simulink model "gm_fourxfour_designfxdpt_givens"  (R2018b)
settings: Solver=FixedStepDiscrete  StartTime=0.0  StopTime=0.18e-6  RelTol=1e-3
InitFcn:
  | if isempty(which('mylib'))
  |      tmp = fileparts(which(bdroot));
  |      run(fullfile(fileparts(tmp), '5-Utilities', 'addPathsPfcHw.m'));
  | end
  | 
  | data_types_givens
StopFcn:
  | GivensSim_Stop
undefined symbols (not defined in the file or in its folder): f
(part 1 of 3)
settings Model: Creator=skanaga4  LastModifiedBy=yangli18
settings OptimizationCC: BlockReduction=off  ConditionallyExecuteInputs=off  DefaultParameterBehavior=Inlined
settings DebuggingCC: AlgebraicLoopMsg=error  ArtificialAlgebraicLoopMsg=none  InheritedTsInSrcMsg=none  SingleTaskRateTransMsg=error
settings HardwareCC: ProdBitPerPointer=32  ProdBitPerSizeT=32  ProdBitPerPtrDiffT=32  ProdLargestAtomicFloat=None  ProdIntDivRoundTo=Undefined  ProdEndianess=Unspecified  ProdWordSize=32  ProdHWDeviceType=ASIC/FPGA->ASIC/FPGA  TargetBitPerLong=64  TargetBitPerPointer=64  TargetBitPerSizeT=64  TargetBitPerPtrDiffT=64  TargetLongLongMode=on  TargetIntDivRoundTo=Zero  TargetEndianess=LittleEndian  TargetWordSize=64  TargetHWDeviceType=Custom Processor->MATLAB Host Computer  ProdEqTarget=off

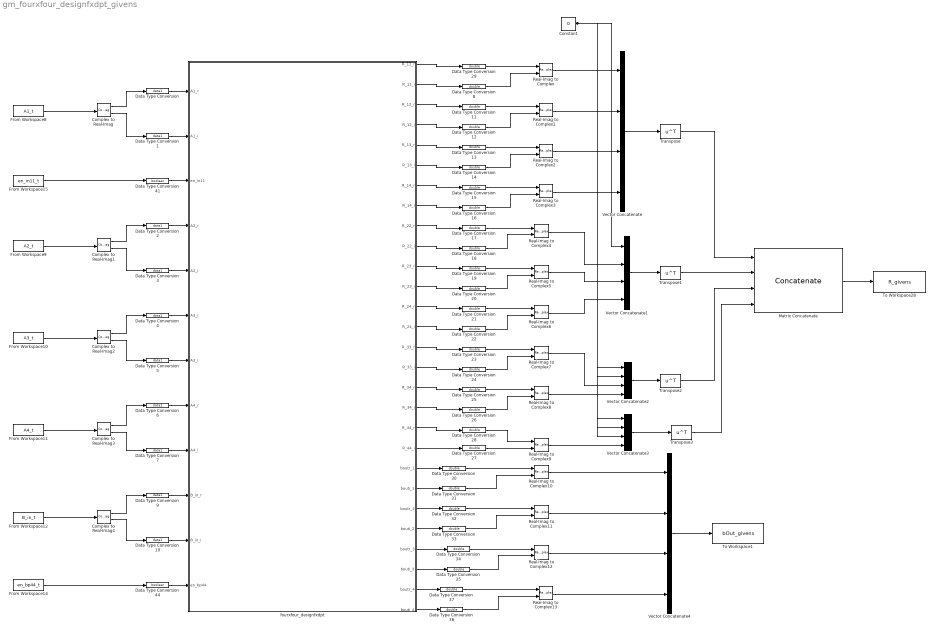
== system gm_fourxfour_designfxdpt_givens ==
  Complex to Real-Imag{,1..4} (5 alike) : ComplexToRealImag
  Constant : Constant  Value=0  SampleTime=-1
  Data Type Conversion{,1..7,9..10} (10 alike) : DataTypeConversion  OutDataTypeStr=data1
  Data Type Conversion{8,11..37} (28 alike) : DataTypeConversion  OutDataTypeStr=double
  Data Type Conversion41 : DataTypeConversion  OutDataTypeStr=boolean
  Data Type Conversion44 : DataTypeConversion  OutDataTypeStr=boolean
  From Workspace10 : FromWorkspace  VariableName=A3_t  SampleTime=1/f  Interpolate=off  OutputAfterFinalValue=Holding final value
  From Workspace11 : FromWorkspace  VariableName=A4_t  SampleTime=1/f  Interpolate=off  OutputAfterFinalValue=Holding final value
  From Workspace12 : FromWorkspace  VariableName=B_in_t  SampleTime=1/f  Interpolate=off  OutputAfterFinalValue=Holding final value
  From Workspace14 : FromWorkspace  VariableName=en_bp44_t  SampleTime=1/f  Interpolate=off  OutputAfterFinalValue=Holding final value
  From Workspace15 : FromWorkspace  VariableName=en_in11_t  SampleTime=1/f  Interpolate=off  OutputAfterFinalValue=Holding final value
  From Workspace8 : FromWorkspace  VariableName=A1_t  SampleTime=1/f  Interpolate=off  OutputAfterFinalValue=Holding final value
  From Workspace9 : FromWorkspace  VariableName=A2_t  SampleTime=1/f  Interpolate=off  OutputAfterFinalValue=Holding final value
  Matrix Concatenate : Concatenate  NumInputs=4  Mode=Multidimensional array
  Real-Imag to Complex{,1..13} (14 alike) : RealImagToComplex
  To Workspace1 : ToWorkspace  VariableName=bOut_givens  SaveFormat=Timeseries  SampleTime=-1
  To Workspace28 : ToWorkspace  VariableName=R_givens  SaveFormat=Timeseries  SampleTime=-1
  Transpose{,1..3} (4 alike) : Math  Operator=transpose  RndMeth=Zero  SaturateOnIntegerOverflow=on
  Vector Concatenate{,1..4} (5 alike) : Concatenate  NumInputs=4
  fourxfour_designfxdpt : Subsystem
  wires:
  Vector Concatenate4/1 -> To Workspace1/1
  Real-Imag to Complex13/1 -> Vector Concatenate4/4
  Real-Imag to Complex12/1 -> Vector Concatenate4/3
  Data Type Conversion30/1 -> Real-Imag to Complex10/1
  Data Type Conversion37/1 -> Real-Imag to Complex13/1
  Data Type Conversion32/1 -> Real-Imag to Complex11/1
  Data Type Conversion33/1 -> Real-Imag to Complex11/2
  Data Type Conversion34/1 -> Real-Imag to Complex12/1
  Real-Imag to Complex11/1 -> Vector Concatenate4/2
  Real-Imag to Complex10/1 -> Vector Concatenate4/1
  Data Type Conversion31/1 -> Real-Imag to Complex10/2
  Data Type Conversion35/1 -> Real-Imag to Complex12/2
  Data Type Conversion36/1 -> Real-Imag to Complex13/2
  fourxfour_designfxdpt/14(R_24_i) -> Data Type Conversion22/1
  fourxfour_designfxdpt/15(R_33_r) -> Data Type Conversion23/1
  fourxfour_designfxdpt/16(R_33_i) -> Data Type Conversion24/1
  fourxfour_designfxdpt/17(R_34_r) -> Data Type Conversion25/1
  fourxfour_designfxdpt/18(R_34_i) -> Data Type Conversion26/1
  Data Type Conversion27/1 -> Real-Imag to Complex9/2
  fourxfour_designfxdpt/19(R_44_r) -> Data Type Conversion28/1
  Real-Imag to Complex3/1 -> Vector Concatenate/4
  Data Type Conversion14/1 -> Real-Imag to Complex2/2
  Real-Imag to Complex1/1 -> Vector Concatenate/2
  Data Type Conversion11/1 -> Real-Imag to Complex1/1
  Data Type Conversion26/1 -> Real-Imag to Complex8/2
  Vector Concatenate2/1 -> Transpose2/1
  Data Type Conversion22/1 -> Real-Imag to Complex6/2
  fourxfour_designfxdpt/10(R_22_i) -> Data Type Conversion18/1
  fourxfour_designfxdpt/1(R_11_r) -> Data Type Conversion29/1
  Transpose1/1 -> Matrix Concatenate/2
  fourxfour_designfxdpt/11(R_23_r) -> Data Type Conversion19/1
  Real-Imag to Complex6/1 -> Vector Concatenate1/4
  Vector Concatenate1/1 -> Transpose1/1
  fourxfour_designfxdpt/20(R_44_i) -> Data Type Conversion27/1
  Data Type Conversion20/1 -> Real-Imag to Complex5/2
  Transpose2/1 -> Matrix Concatenate/3
  Data Type Conversion19/1 -> Real-Imag to Complex5/1
  fourxfour_designfxdpt/8(R_14_i) -> Data Type Conversion16/1
  fourxfour_designfxdpt/13(R_24_r) -> Data Type Conversion21/1
  Transpose3/1 -> Matrix Concatenate/4
  fourxfour_designfxdpt/9(R_22_r) -> Data Type Conversion17/1
  Real-Imag to Complex7/1 -> Vector Concatenate2/3
  fourxfour_designfxdpt/2(R_11_i) -> Data Type Conversion8/1
  Transpose/1 -> Matrix Concatenate/1
  fourxfour_designfxdpt/12(R_23_i) -> Data Type Conversion20/1
  Data Type Conversion25/1 -> Real-Imag to Complex8/1
  Data Type Conversion24/1 -> Real-Imag to Complex7/2
  Data Type Conversion8/1 -> Real-Imag to Complex/2
  Data Type Conversion23/1 -> Real-Imag to Complex7/1
  fourxfour_designfxdpt/7(R_14_r) -> Data Type Conversion15/1
  Vector Concatenate3/1 -> Transpose3/1
  fourxfour_designfxdpt/5(R_13_r) -> Data Type Conversion13/1
  fourxfour_designfxdpt/4(R_12_i) -> Data Type Conversion12/1
  fourxfour_designfxdpt/3(R_12_r) -> Data Type Conversion11/1
  fourxfour_designfxdpt/6(R_13_i) -> Data Type Conversion14/1
  Matrix Concatenate/1 -> To Workspace28/1
  Data Type Conversion29/1 -> Real-Imag to Complex/1
  Data Type Conversion28/1 -> Real-Imag to Complex9/1
  Data Type Conversion15/1 -> Real-Imag to Complex3/1
  Data Type Conversion18/1 -> Real-Imag to Complex4/2
  Data Type Conversion17/1 -> Real-Imag to Complex4/1
  Data Type Conversion16/1 -> Real-Imag to Complex3/2
  Data Type Conversion12/1 -> Real-Imag to Complex1/2
  Data Type Conversion13/1 -> Real-Imag to Complex2/1
  Data Type Conversion21/1 -> Real-Imag to Complex6/1
  Real-Imag to Complex5/1 -> Vector Concatenate1/3
  Vector Concatenate/1 -> Transpose/1
  Real-Imag to Complex2/1 -> Vector Concatenate/3
  Real-Imag to Complex8/1 -> Vector Concatenate2/4
  Real-Imag to Complex9/1 -> Vector Concatenate3/4
  Real-Imag to Complex4/1 -> Vector Concatenate1/2
  Constant/1 -> Vector Concatenate1/1, Vector Concatenate2/1, Vector Concatenate2/2, Vector Concatenate3/1, Vector Concatenate3/2, Vector Concatenate3/3
  Real-Imag to Complex/1 -> Vector Concatenate/1
  From Workspace15/1 -> Data Type Conversion41/1
  From Workspace14/1 -> Data Type Conversion44/1
  Complex to Real-Imag4/2 -> Data Type Conversion10/1
  Complex to Real-Imag4/1 -> Data Type Conversion9/1
  From Workspace12/1 -> Complex to Real-Imag4/1
  Complex to Real-Imag3/2 -> Data Type Conversion7/1
  Complex to Real-Imag3/1 -> Data Type Conversion6/1
  Complex to Real-Imag2/2 -> Data Type Conversion5/1
  Complex to Real-Imag2/1 -> Data Type Conversion4/1
  Complex to Real-Imag1/2 -> Data Type Conversion3/1
  Complex to Real-Imag1/1 -> Data Type Conversion2/1
  From Workspace10/1 -> Complex to Real-Imag2/1
  From Workspace11/1 -> Complex to Real-Imag3/1
  From Workspace9/1 -> Complex to Real-Imag1/1
  Complex to Real-Imag/2 -> Data Type Conversion1/1
  Complex to Real-Imag/1 -> Data Type Conversion/1
  From Workspace8/1 -> Complex to Real-Imag/1
  Data Type Conversion10/1 -> fourxfour_designfxdpt/11(B_in_i)
  Data Type Conversion9/1 -> fourxfour_designfxdpt/10(B_in_r)
  fourxfour_designfxdpt/26(bouti_3) -> Data Type Conversion35/1
  fourxfour_designfxdpt/25(boutr_3) -> Data Type Conversion34/1
  fourxfour_designfxdpt/27(boutr_4) -> Data Type Conversion37/1
  fourxfour_designfxdpt/28(bouti_4) -> Data Type Conversion36/1
  fourxfour_designfxdpt/23(boutr_2) -> Data Type Conversion32/1
  fourxfour_designfxdpt/24(bouti_2) -> Data Type Conversion33/1
  fourxfour_designfxdpt/22(bouti_1) -> Data Type Conversion31/1
  fourxfour_designfxdpt/21(boutr_1) -> Data Type Conversion30/1
  Data Type Conversion44/1 -> fourxfour_designfxdpt/12(en_bp44)
  Data Type Conversion41/1 -> fourxfour_designfxdpt/3("en_in11 ")
  Data Type Conversion7/1 -> fourxfour_designfxdpt/9(A4_i)
  Data Type Conversion6/1 -> fourxfour_designfxdpt/8(A4_r)
  Data Type Conversion5/1 -> fourxfour_designfxdpt/7(A3_i)
  Data Type Conversion4/1 -> fourxfour_designfxdpt/6(A3_r)
  Data Type Conversion3/1 -> fourxfour_designfxdpt/5(A2_i)
  Data Type Conversion2/1 -> fourxfour_designfxdpt/4(A2_r)
  Data Type Conversion1/1 -> fourxfour_designfxdpt/2(A1_i)
  Data Type Conversion/1 -> fourxfour_designfxdpt/1("A1_r ")

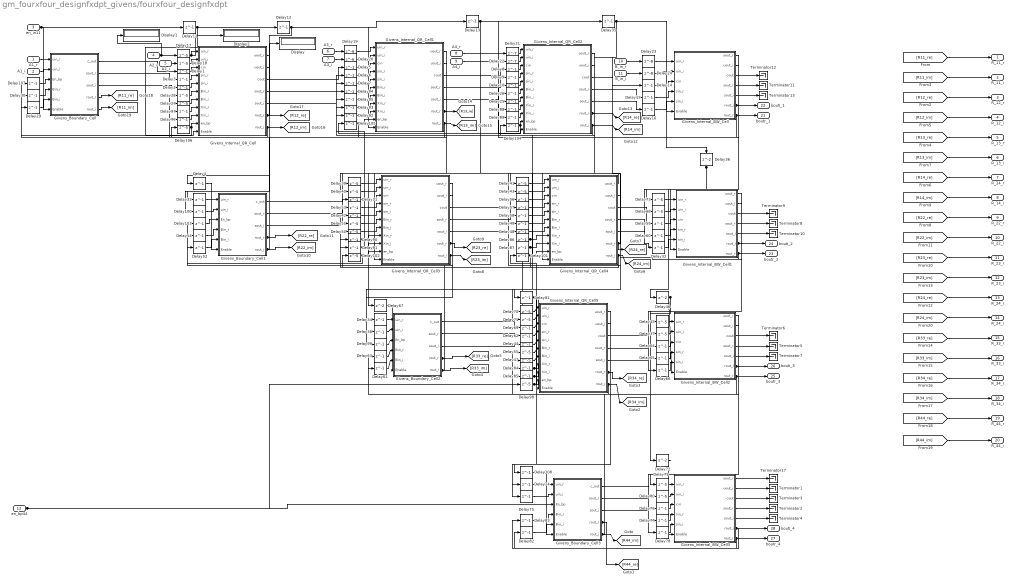
== system gm_fourxfour_designfxdpt_givens/fourxfour_designfxdpt ==
  "A1_r " : Inport  OutDataTypeStr=fixdt(1, 24, 14)  PortDimensions=1  SampleTime=1e-08
  A1_i : Inport  Port=2  OutDataTypeStr=fixdt(1, 24, 14)  PortDimensions=1  SampleTime=1e-08
  "en_in11 " : Inport  Port=3  OutDataTypeStr=boolean  PortDimensions=1  SampleTime=1e-08
  A2_r : Inport  Port=4  OutDataTypeStr=fixdt(1, 24, 14)  PortDimensions=1  SampleTime=1e-08
  A2_i : Inport  Port=5  OutDataTypeStr=fixdt(1, 24, 14)  PortDimensions=1  SampleTime=1e-08
  A3_r : Inport  Port=6  OutDataTypeStr=fixdt(1, 24, 14)  PortDimensions=1  SampleTime=1e-08
  A3_i : Inport  Port=7  OutDataTypeStr=fixdt(1, 24, 14)  PortDimensions=1  SampleTime=1e-08
  A4_r : Inport  Port=8  OutDataTypeStr=fixdt(1, 24, 14)  PortDimensions=1  SampleTime=1e-08
  A4_i : Inport  Port=9  OutDataTypeStr=fixdt(1, 24, 14)  PortDimensions=1  SampleTime=1e-08
  B_in_r : Inport  Port=10  OutDataTypeStr=fixdt(1, 24, 14)  PortDimensions=1  SampleTime=1e-08
  B_in_i : Inport  Port=11  OutDataTypeStr=fixdt(1, 24, 14)  PortDimensions=1  SampleTime=1e-08
  en_bp44 : Inport  Port=12  OutDataTypeStr=boolean  PortDimensions=1  SampleTime=1e-08
  Delay{1..16,25..26,29..35,38,42,44,48..49,52..54,56..66,69,74..78,81..97,99..101,103..105,107..108} (75 alike) : Delay  DelayLength=1  InitialCondition=0
  Delay{17..18,27..28,37,39..41,43,45,47,50..51,55,68,70..71,73,79..80,98,102,106} (23 alike) : Delay  DelayLength=5  InitialCondition=0
  Delay19 : Delay  DelayLength=6  InitialCondition=0
  Delay20 : Delay  DelayLength=6  InitialCondition=0
  Delay21 : Delay  DelayLength=7  InitialCondition=0
  Delay22 : Delay  DelayLength=7  InitialCondition=0
  Delay23 : Delay  DelayLength=8  InitialCondition=0
  Delay24 : Delay  DelayLength=8  InitialCondition=0
  Delay{36,46,67,72} (4 alike) : Delay  InitialCondition=0
  Display : Display
  Display1 : Display
  Display2 : Display
  Givens_Boundary_Cell : Subsystem
  Givens_Boundary_Cell1 : Subsystem
  Givens_Boundary_Cell2 : Subsystem
  Givens_Boundary_Cell3 : Subsystem
  Givens_Internal_BW_Cell : Subsystem
  Givens_Internal_BW_Cell1 : Subsystem
  Givens_Internal_BW_Cell2 : Subsystem
  Givens_Internal_BW_Cell3 : Subsystem
  Givens_Internal_QR_Cell : Subsystem
  Givens_Internal_QR_Cell1 : Subsystem
  Givens_Internal_QR_Cell2 : Subsystem
  Givens_Internal_QR_Cell3 : Subsystem
  Givens_Internal_QR_Cell4 : Subsystem
  Givens_Internal_QR_Cell5 : Subsystem
  Terminator{1..13,17} (14 alike) : Terminator
  R_11_r : Outport
  R_11_i : Outport  Port=2
  R_12_r : Outport  Port=3
  R_12_i : Outport  Port=4
  R_13_r : Outport  Port=5
  R_13_i : Outport  Port=6
  R_14_r : Outport  Port=7
  R_14_i : Outport  Port=8
  R_22_r : Outport  Port=9
  R_22_i : Outport  Port=10
  R_23_r : Outport  Port=11
  R_23_i : Outport  Port=12
  R_24_r : Outport  Port=13
  R_24_i : Outport  Port=14
  R_33_r : Outport  Port=15
  R_33_i : Outport  Port=16
  R_34_r : Outport  Port=17
  R_34_i : Outport  Port=18
  R_44_r : Outport  Port=19
  R_44_i : Outport  Port=20
  boutr_1 : Outport  Port=21
  bouti_1 : Outport  Port=22
  boutr_2 : Outport  Port=23
  bouti_2 : Outport  Port=24
  boutr_3 : Outport  Port=25
  bouti_3 : Outport  Port=26
  boutr_4 : Outport  Port=27
  bouti_4 : Outport  Port=28
  wires:
  "A1_r "/1 -> Givens_Boundary_Cell/1(uin_r)
  A1_i/1 -> Givens_Boundary_Cell/2(uin_i)
  "en_in11 "/1 -> Delay11/1, Givens_Boundary_Cell/6(Enable)
  A2_r/1 -> Display1/1, Delay17/1
  A2_i/1 -> Delay18/1
  A3_r/1 -> Delay19/1
  A3_i/1 -> Delay20/1
  A4_r/1 -> Delay21/1
  A4_i/1 -> Delay22/1
  B_in_r/1 -> Delay23/1
  B_in_i/1 -> Delay24/1
  en_bp44/1 -> Delay98/1, Givens_Boundary_Cell3/3(En_bp)
  Delay101/1 -> Delay104/1, Delay102/1, Givens_Internal_QR_Cell4/10(en_bp)
  Delay102/1 -> Delay103/1, Givens_Internal_QR_Cell3/10(en_bp)
  Delay103/1 -> Givens_Boundary_Cell1/3(En_bp)
  Delay104/1 -> Delay105/1, Givens_Internal_QR_Cell2/10(en_bp)
  Delay105/1 -> Delay106/1, Givens_Internal_QR_Cell1/10(en_bp)
  Delay106/1 -> Delay107/1, Givens_Internal_QR_Cell/10(en_bp)
  Delay107/1 -> Givens_Boundary_Cell/3(En_bp)
  Delay108/1 -> Givens_Boundary_Cell3/6(Enable)
  Delay11/1 -> Delay12/1, Givens_Internal_QR_Cell/11(Enable)
  Delay12/1 -> Delay4/1, Delay13/1, Givens_Internal_QR_Cell1/11(Enable)
  Delay13/1 -> Delay35/1, Givens_Internal_QR_Cell2/11(Enable), Givens_Internal_QR_Cell3/11(Enable)
  Delay17/1 -> Display2/1, Givens_Internal_QR_Cell/1(uin_r)
  Delay18/1 -> Givens_Internal_QR_Cell/2(uin_i)
  Delay19/1 -> Givens_Internal_QR_Cell1/1(uin_r)
  Delay20/1 -> Givens_Internal_QR_Cell1/2(uin_i)
  Delay21/1 -> Givens_Internal_QR_Cell2/1(uin_r)
  Delay22/1 -> Givens_Internal_QR_Cell2/2(uin_i)
  Delay23/1 -> Givens_Internal_BW_Cell/1(uin_r)
  Delay24/1 -> Givens_Internal_BW_Cell/2(uin_i)
  Delay35/1 -> Delay81/1, Delay67/1, Delay36/1, Givens_Internal_QR_Cell4/11(Enable), Givens_Internal_BW_Cell/6(Enable)
  Delay36/1 -> Delay46/1, Givens_Internal_BW_Cell1/6(Enable)
  Delay4/1 -> Givens_Boundary_Cell1/6(Enable)
  Delay46/1 -> Delay72/1, Givens_Internal_BW_Cell2/6(Enable)
  Delay67/1 -> Givens_Boundary_Cell2/6(Enable)
  Delay72/1 -> Givens_Internal_BW_Cell3/6(Enable)
  Delay81/1 -> Delay108/1, Givens_Internal_QR_Cell5/11(Enable)
  Delay98/1 -> Delay99/1, Delay101/1, Givens_Internal_QR_Cell5/10(en_bp)
  Delay99/1 -> Givens_Boundary_Cell2/3(En_bp)
  [R11_re] -> R_11_r/1
  [R23_re] -> R_23_r/1
  [R22_im] -> R_22_i/1
  [R24_re] -> R_24_r/1
  [R23_im] -> R_23_i/1
  [R33_re] -> R_33_r/1
  [R33_im] -> R_33_i/1
  [R34_re] -> R_34_r/1
  [R34_im] -> R_34_i/1
  [R44_re] -> R_44_r/1
  [R44_im] -> R_44_i/1
  [R12_re] -> R_12_r/1
  [R24_im] -> R_24_i/1
  [R11_im] -> R_11_i/1
  [R13_re] -> R_13_r/1
  [R12_im] -> R_12_i/1
  [R14_re] -> R_14_r/1
  [R13_im] -> R_13_i/1
  [R22_re] -> R_22_r/1
  [R14_im] -> R_14_i/1
  Givens_Boundary_Cell/4(rout_r) -> [R11_re]
  Givens_Boundary_Cell/5(rout_i) -> [R11_im]
  Givens_Boundary_Cell1/4(rout_r) -> [R22_re], Delay97/1
  Givens_Boundary_Cell1/5(rout_i) -> [R22_im], Delay96/1
  Givens_Boundary_Cell2/4(rout_r) -> [R33_re], Delay90/1
  Givens_Boundary_Cell2/5(rout_i) -> [R33_im], Delay91/1
  Givens_Boundary_Cell3/4(rout_r) -> [R44_re], Delay84/1
  Givens_Boundary_Cell3/5(rout_i) -> [R44_im], Delay85/1
  Givens_Internal_BW_Cell/3(cout) -> Terminator12/1
  Givens_Internal_BW_Cell/4(sout_r) -> Terminator11/1
  Givens_Internal_BW_Cell/5(sout_i) -> Terminator13/1
  Givens_Internal_BW_Cell/6(rout_i) -> bouti_1/1, Delay25/1
  Givens_Internal_BW_Cell/7(rout_r) -> boutr_1/1, Delay26/1
  Givens_Internal_BW_Cell1/3(cout) -> Terminator9/1
  Givens_Internal_BW_Cell1/4(sout_r) -> Terminator8/1
  Givens_Internal_BW_Cell1/5(sout_i) -> Terminator10/1
  Givens_Internal_BW_Cell1/6(rout_i) -> bouti_2/1, Delay48/1
  Givens_Internal_BW_Cell1/7(rout_r) -> boutr_2/1, Delay49/1
  Givens_Internal_BW_Cell2/3(cout) -> Terminator6/1
  Givens_Internal_BW_Cell2/4(sout_r) -> Terminator5/1
  Givens_Internal_BW_Cell2/5(sout_i) -> Terminator7/1
  Givens_Internal_BW_Cell2/6(rout_i) -> bouti_3/1, Delay47/1
  Givens_Internal_BW_Cell2/7(rout_r) -> boutr_3/1, Delay55/1
  Givens_Internal_BW_Cell3/1(uout_r) -> Terminator17/1
  Givens_Internal_BW_Cell3/2(uout_i) -> Terminator1/1
  Givens_Internal_BW_Cell3/3(cout) -> Terminator3/1
  Givens_Internal_BW_Cell3/4(sout_r) -> Terminator2/1
  Givens_Internal_BW_Cell3/5(sout_i) -> Terminator4/1
  Givens_Internal_BW_Cell3/6(rout_i) -> bouti_4/1, Delay82/1
  Givens_Internal_BW_Cell3/7(rout_r) -> boutr_4/1, Delay83/1
  Givens_Internal_QR_Cell/6(rout_r) -> [R12_re], Display/1, Delay30/1
  Givens_Internal_QR_Cell/7(rout_i) -> [R12_im], Delay29/1
  Givens_Internal_QR_Cell1/6(rout_r) -> [R13_re], Delay28/1
  Givens_Internal_QR_Cell1/7(rout_i) -> [R13_im], Delay27/1
  Givens_Internal_QR_Cell2/6(rout_r) -> [R14_re], Delay94/1
  Givens_Internal_QR_Cell2/7(rout_i) -> [R14_im], Delay95/1
  Givens_Internal_QR_Cell3/6(rout_r) -> [R23_re], Delay54/1
  Givens_Internal_QR_Cell3/7(rout_i) -> [R23_im], Delay52/1
  Givens_Internal_QR_Cell4/6(rout_r) -> [R24_re], Delay51/1
  Givens_Internal_QR_Cell4/7(rout_i) -> [R24_im], Delay50/1
  Givens_Internal_QR_Cell5/6(rout_r) -> [R34_re], Delay63/1
  Givens_Internal_QR_Cell5/7(rout_i) -> [R34_im], Delay61/1
  Delay29/1 -> Givens_Boundary_Cell/5(Bin_i)
  Delay30/1 -> Givens_Boundary_Cell/4(Bin_r)
  Delay96/1 -> Givens_Internal_QR_Cell/9(Xin_i)
  Delay97/1 -> Givens_Internal_QR_Cell/8(Xin_r)
  Delay27/1 -> Givens_Internal_QR_Cell/7(Bin_i)
  Delay28/1 -> Givens_Internal_QR_Cell/6(Bin_r)
  Delay92/1 -> Givens_Internal_QR_Cell1/9(Xin_i)
  Delay93/1 -> Givens_Internal_QR_Cell1/8(Xin_r)
  Delay95/1 -> Givens_Internal_QR_Cell1/7(Bin_i)
  Delay94/1 -> Givens_Internal_QR_Cell1/6(Bin_r)
  Delay89/1 -> Givens_Internal_QR_Cell2/9(Xin_i)
  Delay88/1 -> Givens_Internal_QR_Cell2/8(Xin_r)
  Delay82/1 -> Givens_Boundary_Cell3/5(Bin_i)
  Delay83/1 -> Givens_Boundary_Cell3/4(Bin_r)
  Delay78/1 -> Givens_Internal_BW_Cell3/5(sin_i)
  Delay77/1 -> Givens_Internal_BW_Cell3/4(sin_r)
  Delay76/1 -> Givens_Internal_BW_Cell3/3(cin)
  Delay80/1 -> Givens_Internal_BW_Cell3/2(uin_i)
  Delay79/1 -> Givens_Internal_BW_Cell3/1(uin_r)
  Delay75/1 -> Givens_Boundary_Cell3/2(uin_i)
  Delay74/1 -> Givens_Boundary_Cell3/1(uin_r)
  Delay47/1 -> Givens_Internal_QR_Cell5/7(Bin_i)
  Delay55/1 -> Givens_Internal_QR_Cell5/6(Bin_r)
  Delay66/1 -> Givens_Internal_BW_Cell2/5(sin_i)
  Delay65/1 -> Givens_Internal_BW_Cell2/4(sin_r)
  Delay64/1 -> Givens_Internal_BW_Cell2/3(cin)
  Delay37/1 -> Givens_Internal_BW_Cell2/2(uin_i)
  Delay45/1 -> Givens_Internal_BW_Cell2/1(uin_r)
  Givens_Internal_BW_Cell2/1(uout_r) -> Delay79/1
  Givens_Internal_BW_Cell2/2(uout_i) -> Delay80/1
  Delay44/1 -> Givens_Internal_QR_Cell5/5(sin_i)
  Delay62/1 -> Givens_Internal_QR_Cell5/4(sin_r)
  Delay69/1 -> Givens_Internal_QR_Cell5/3(cin)
  Delay71/1 -> Givens_Internal_QR_Cell5/2(uin_i)
  Delay70/1 -> Givens_Internal_QR_Cell5/1(uin_r)
  Delay87/1 -> Delay89/1, Givens_Internal_QR_Cell4/9(Xin_i)
  Delay85/1 -> Delay87/1, Givens_Internal_QR_Cell5/9(Xin_i)
  Delay84/1 -> Delay86/1, Givens_Internal_QR_Cell5/8(Xin_r)
  Delay86/1 -> Delay88/1, Givens_Internal_QR_Cell4/8(Xin_r)
  Delay48/1 -> Givens_Internal_QR_Cell4/7(Bin_i)
  Delay49/1 -> Givens_Internal_QR_Cell4/6(Bin_r)
  Delay32/1 -> Givens_Internal_BW_Cell1/5(sin_i)
  Delay60/1 -> Givens_Internal_BW_Cell1/4(sin_r)
  Delay59/1 -> Givens_Internal_BW_Cell1/3(cin)
  Delay68/1 -> Givens_Internal_BW_Cell1/2(uin_i)
  Delay73/1 -> Givens_Internal_BW_Cell1/1(uin_r)
  Givens_Internal_BW_Cell1/1(uout_r) -> Delay45/1
  Givens_Internal_BW_Cell1/2(uout_i) -> Delay37/1
  Delay58/1 -> Givens_Internal_QR_Cell4/5(sin_i)
  Delay57/1 -> Givens_Internal_QR_Cell4/4(sin_r)
  Delay56/1 -> Givens_Internal_QR_Cell4/3(cin)
  Delay91/1 -> Delay92/1, Givens_Internal_QR_Cell3/9(Xin_i)
  Delay90/1 -> Delay93/1, Givens_Internal_QR_Cell3/8(Xin_r)
  Delay61/1 -> Givens_Boundary_Cell2/5(Bin_i)
  Delay63/1 -> Givens_Boundary_Cell2/4(Bin_r)
  Delay38/1 -> Givens_Boundary_Cell2/2(uin_i)
  Delay34/1 -> Givens_Boundary_Cell2/1(uin_r)
  Givens_Boundary_Cell2/1(c_out) -> Delay69/1
  Givens_Boundary_Cell2/2(sout_r) -> Delay62/1
  Givens_Boundary_Cell2/3(sout_i) -> Delay44/1
  Delay50/1 -> Givens_Internal_QR_Cell3/7(Bin_i)
  Delay51/1 -> Givens_Internal_QR_Cell3/6(Bin_r)
  Delay42/1 -> Givens_Internal_QR_Cell3/5(sin_i)
  Delay53/1 -> Givens_Internal_QR_Cell3/4(sin_r)
  Delay31/1 -> Givens_Internal_QR_Cell3/3(cin)
  Delay52/1 -> Givens_Boundary_Cell1/5(Bin_i)
  Delay54/1 -> Givens_Boundary_Cell1/4(Bin_r)
  Delay100/1 -> Givens_Boundary_Cell1/2(uin_i)
  Delay33/1 -> Givens_Boundary_Cell1/1(uin_r)
  Givens_Boundary_Cell1/1(c_out) -> Delay31/1
  Givens_Boundary_Cell1/2(sout_r) -> Delay53/1
  Givens_Boundary_Cell1/3(sout_i) -> Delay42/1
  Delay40/1 -> Givens_Internal_QR_Cell3/2(uin_i)
  Delay39/1 -> Givens_Internal_QR_Cell3/1(uin_r)
  Givens_Internal_QR_Cell3/1(uout_r) -> Delay34/1
  Givens_Internal_QR_Cell3/2(uout_i) -> Delay38/1
  Givens_Internal_QR_Cell3/3(cout) -> Delay56/1
  Givens_Internal_QR_Cell3/4(sout_r) -> Delay57/1
  Givens_Internal_QR_Cell3/5(sout_i) -> Delay58/1
  Delay43/1 -> Givens_Internal_QR_Cell4/2(uin_i)
  Delay41/1 -> Givens_Internal_QR_Cell4/1(uin_r)
  Givens_Internal_QR_Cell4/1(uout_r) -> Delay70/1
  Givens_Internal_QR_Cell4/2(uout_i) -> Delay71/1
  Givens_Internal_QR_Cell4/3(cout) -> Delay59/1
  Givens_Internal_QR_Cell4/4(sout_r) -> Delay60/1
  Givens_Internal_QR_Cell4/5(sout_i) -> Delay32/1
  Givens_Internal_QR_Cell5/1(uout_r) -> Delay74/1
  Givens_Internal_QR_Cell5/2(uout_i) -> Delay75/1
  Givens_Internal_QR_Cell5/3(cout) -> Delay64/1
  Givens_Internal_QR_Cell5/4(sout_r) -> Delay65/1
  Givens_Internal_QR_Cell5/5(sout_i) -> Delay66/1
  Givens_Boundary_Cell3/1(c_out) -> Delay76/1
  Givens_Boundary_Cell3/2(sout_r) -> Delay77/1
  Givens_Boundary_Cell3/3(sout_i) -> Delay78/1
  Delay25/1 -> Givens_Internal_QR_Cell2/7(Bin_i)
  Delay26/1 -> Givens_Internal_QR_Cell2/6(Bin_r)
  Delay16/1 -> Givens_Internal_BW_Cell/5(sin_i)
  Delay15/1 -> Givens_Internal_BW_Cell/4(sin_r)
  Delay14/1 -> Givens_Internal_BW_Cell/3(cin)
  Givens_Internal_BW_Cell/1(uout_r) -> Delay73/1
  Givens_Internal_BW_Cell/2(uout_i) -> Delay68/1
  Delay10/1 -> Givens_Internal_QR_Cell2/5(sin_i)
  Delay9/1 -> Givens_Internal_QR_Cell2/4(sin_r)
  Delay8/1 -> Givens_Internal_QR_Cell2/3(cin)
  Givens_Internal_QR_Cell2/1(uout_r) -> Delay41/1
  Givens_Internal_QR_Cell2/2(uout_i) -> Delay43/1
  Givens_Internal_QR_Cell2/3(cout) -> Delay14/1
  Givens_Internal_QR_Cell2/4(sout_r) -> Delay15/1
  Givens_Internal_QR_Cell2/5(sout_i) -> Delay16/1
  Delay7/1 -> Givens_Internal_QR_Cell1/5(sin_i)
  Delay6/1 -> Givens_Internal_QR_Cell1/4(sin_r)
  Delay5/1 -> Givens_Internal_QR_Cell1/3(cin)
  Givens_Internal_QR_Cell1/1(uout_r) -> Delay39/1
  Givens_Internal_QR_Cell1/2(uout_i) -> Delay40/1
  Givens_Internal_QR_Cell1/3(cout) -> Delay8/1
  Givens_Internal_QR_Cell1/4(sout_r) -> Delay9/1
  Givens_Internal_QR_Cell1/5(sout_i) -> Delay10/1
  Delay2/1 -> Givens_Internal_QR_Cell/5(sin_i)
  Delay3/1 -> Givens_Internal_QR_Cell/4(sin_r)
  Delay1/1 -> Givens_Internal_QR_Cell/3(cin)
  Givens_Internal_QR_Cell/1(uout_r) -> Delay33/1
  Givens_Internal_QR_Cell/2(uout_i) -> Delay100/1
  Givens_Internal_QR_Cell/3(cout) -> Delay5/1
  Givens_Internal_QR_Cell/4(sout_r) -> Delay6/1
  Givens_Internal_QR_Cell/5(sout_i) -> Delay7/1
  Givens_Boundary_Cell/1(c_out) -> Delay1/1
  Givens_Boundary_Cell/2(sout_r) -> Delay3/1
  Givens_Boundary_Cell/3(sout_i) -> Delay2/1

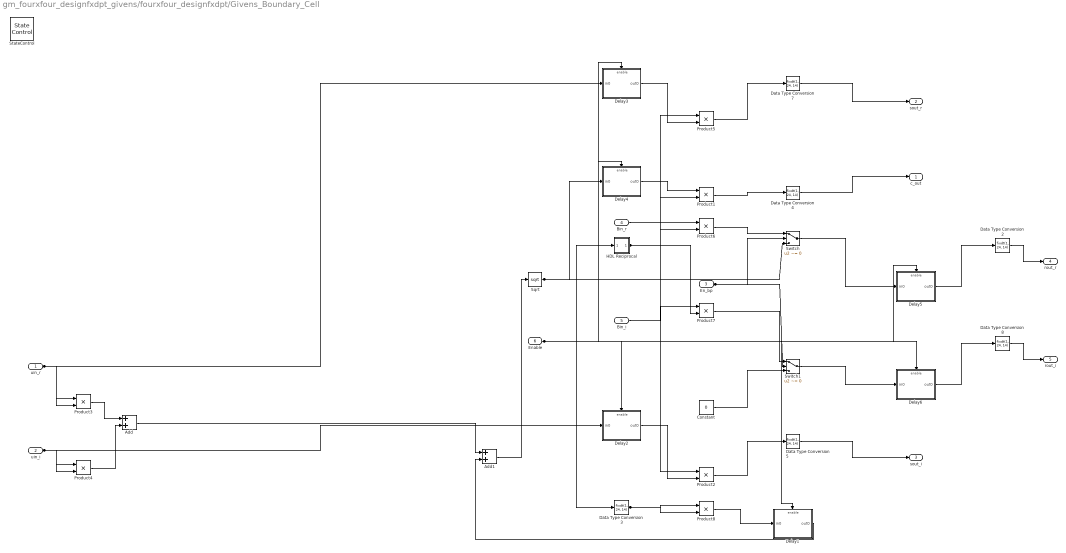
== system gm_fourxfour_designfxdpt_givens/fourxfour_designfxdpt/Givens_Boundary_Cell ==
  uin_r : Inport  OutDataTypeStr=fixdt(1, 24, 14)  SampleTime=1e-08
  uin_i : Inport  Port=2  OutDataTypeStr=fixdt(1, 24, 14)  SampleTime=1e-08
  En_bp : Inport  Port=3  OutDataTypeStr=boolean  SampleTime=1e-08
  Bin_r : Inport  Port=4  OutDataTypeStr=fixdt(1, 24, 14)  SampleTime=1e-08
  Bin_i : Inport  Port=5  OutDataTypeStr=fixdt(1, 24, 14)  SampleTime=1e-08
  Enable : Inport  Port=6  OutDataTypeStr=boolean  SampleTime=1e-08
  Add : Sum  AccumDataTypeStr=fixdt(1, 49, 28)  OutDataTypeStr=fixdt(1, 49, 28)  SampleTime=1e-08
  Add1 : Sum  AccumDataTypeStr=fixdt(1, 50, 28)  OutDataTypeStr=fixdt(0, 49, 28)  SampleTime=1e-08
  Constant : Constant  Value=0  OutDataTypeStr=fixdt(1, 24, 14)  SampleTime=-1
  Data Type Conversion{2..5,7..8} (6 alike) : DataTypeConversion  OutDataTypeStr=fixdt(1, 24, 14)  SampleTime=1e-08
  Delay1 : Subsystem
      settings: MinAlgLoopOccurrences=on
  Delay2 : Subsystem
      settings: MinAlgLoopOccurrences=on
  Delay3 : Subsystem
      settings: MinAlgLoopOccurrences=on
  Delay4 : Subsystem
      settings: MinAlgLoopOccurrences=on
  Delay5 : Subsystem
      settings: MinAlgLoopOccurrences=on
  Delay6 : Subsystem
      settings: MinAlgLoopOccurrences=on
  HDL Reciprocal : Subsystem
  Product1 : Product  Inputs=**  OutDataTypeStr=fixdt(0, 98, 48)  SampleTime=1e-08
  Product{2,5..7} (4 alike) : Product  Inputs=**  OutDataTypeStr=fixdt(1, 73, 34)  SampleTime=1e-08
  Product3 : Product  Inputs=**  OutDataTypeStr=fixdt(1, 48, 28)  SampleTime=1e-08
  Product4 : Product  Inputs=**  OutDataTypeStr=fixdt(1, 48, 28)  SampleTime=1e-08
  Product8 : Product  Inputs=**  OutDataTypeStr=fixdt(1, 48, 28)  SampleTime=1e-08
  Sqrt : Sqrt  OutputSignalType=real  SaturateOnIntegerOverflow=on
  StateControl : StateControl  StateControl=Synchronous
  Switch : Switch  Criteria=u2 ~= 0  Threshold=double(0)  OutDataTypeStr=fixdt(1, 73, 34)  SampleTime=1e-08
  Switch1 : Switch  Criteria=u2 ~= 0  Threshold=double(0)  OutDataTypeStr=fixdt(1, 73, 34)  SampleTime=1e-08
  c_out : Outport  InitialOutput=0
  sout_r : Outport  Port=2  InitialOutput=0
  sout_i : Outport  Port=3  InitialOutput=0
  rout_r : Outport  Port=4  InitialOutput=0
  rout_i : Outport  Port=5  InitialOutput=0
  wires:
  Enable/1 -> Delay6/Enable, Delay5/Enable, Delay4/Enable, Delay3/Enable, Delay2/Enable, Delay1/Enable
  uin_r/1 -> Product3/2, Product3/1, Delay3/1(in0)
  uin_i/1 -> Product4/2, Product4/1, Delay2/1(in0)
  En_bp/1 -> Switch1/2, Switch/2
  Bin_r/1 -> Product6/1
  Bin_i/1 -> Product7/1
  Add/1 -> Add1/1
  Add1/1 -> Sqrt/1
  Constant/1 -> Switch1/3
  Data Type Conversion2/1 -> rout_r/1
  Data Type Conversion3/1 -> Product8/2, Product8/1
  Data Type Conversion4/1 -> c_out/1
  Data Type Conversion5/1 -> sout_i/1
  Data Type Conversion7/1 -> sout_r/1
  Data Type Conversion8/1 -> rout_i/1
  Delay1/1(out0) -> Add1/2
  Delay2/1(out0) -> Product2/2
  Delay3/1(out0) -> Product5/2
  Delay4/1(out0) -> Product1/1
  Delay5/1(out0) -> Data Type Conversion2/1
  Delay6/1(out0) -> Data Type Conversion8/1
  HDL Reciprocal/1(Out1) -> Product7/2, Product6/2, Product5/1, Product2/1, Product1/2
  Product1/1 -> Data Type Conversion4/1
  Product2/1 -> Data Type Conversion5/1
  Product3/1 -> Add/1
  Product4/1 -> Add/2
  Product5/1 -> Data Type Conversion7/1
  Product6/1 -> Switch/1
  Product7/1 -> Switch1/1
  Product8/1 -> Delay1/1(in0)
  Sqrt/1 -> Switch/3, HDL Reciprocal/1(In1), Data Type Conversion3/1, Delay4/1(in0)
  Switch/1 -> Delay5/1(in0)
  Switch1/1 -> Delay6/1(in0)

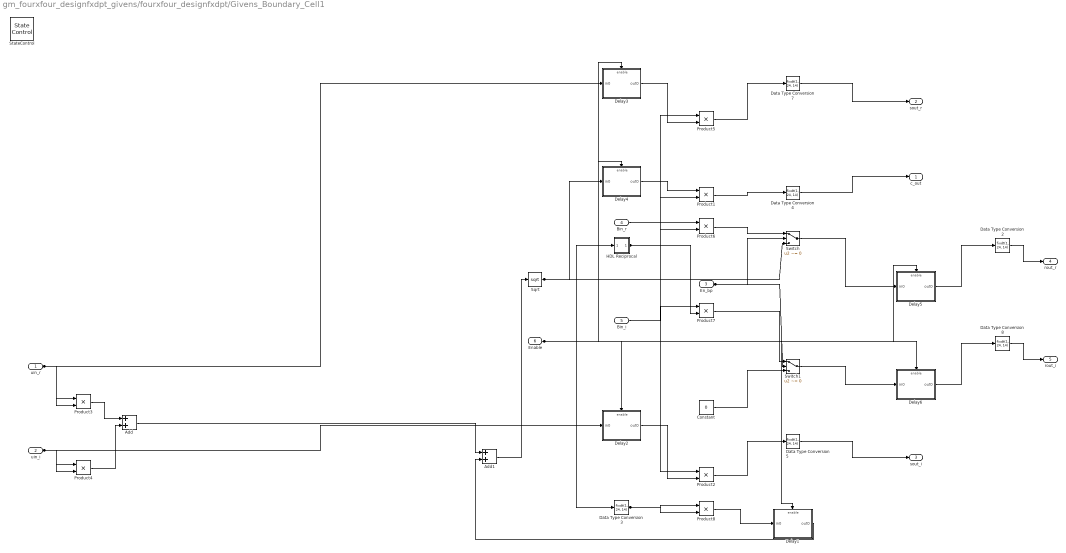
== system gm_fourxfour_designfxdpt_givens/fourxfour_designfxdpt/Givens_Boundary_Cell1 ==
  uin_r : Inport  OutDataTypeStr=fixdt(1, 24, 14)  SampleTime=1e-08
  uin_i : Inport  Port=2  OutDataTypeStr=fixdt(1, 24, 14)  SampleTime=1e-08
  En_bp : Inport  Port=3  OutDataTypeStr=boolean  SampleTime=1e-08
  Bin_r : Inport  Port=4  OutDataTypeStr=fixdt(1, 24, 14)  SampleTime=1e-08
  Bin_i : Inport  Port=5  OutDataTypeStr=fixdt(1, 24, 14)  SampleTime=1e-08
  Enable : Inport  Port=6  OutDataTypeStr=boolean  SampleTime=1e-08
  Add : Sum  AccumDataTypeStr=fixdt(1, 49, 28)  OutDataTypeStr=fixdt(1, 49, 28)  SampleTime=1e-08
  Add1 : Sum  AccumDataTypeStr=fixdt(1, 50, 28)  OutDataTypeStr=fixdt(0, 49, 28)  SampleTime=1e-08
  Constant : Constant  Value=0  OutDataTypeStr=fixdt(1, 24, 14)  SampleTime=-1
  Data Type Conversion{2..5,7..8} (6 alike) : DataTypeConversion  OutDataTypeStr=fixdt(1, 24, 14)  SampleTime=1e-08
  Delay1 : Subsystem
      settings: MinAlgLoopOccurrences=on
  Delay2 : Subsystem
      settings: MinAlgLoopOccurrences=on
  Delay3 : Subsystem
      settings: MinAlgLoopOccurrences=on
  Delay4 : Subsystem
      settings: MinAlgLoopOccurrences=on
  Delay5 : Subsystem
      settings: MinAlgLoopOccurrences=on
  Delay6 : Subsystem
      settings: MinAlgLoopOccurrences=on
  HDL Reciprocal : Subsystem
  Product1 : Product  Inputs=**  OutDataTypeStr=fixdt(0, 98, 48)  SampleTime=1e-08
  Product{2,5..7} (4 alike) : Product  Inputs=**  OutDataTypeStr=fixdt(1, 73, 34)  SampleTime=1e-08
  Product3 : Product  Inputs=**  OutDataTypeStr=fixdt(1, 48, 28)  SampleTime=1e-08
  Product4 : Product  Inputs=**  OutDataTypeStr=fixdt(1, 48, 28)  SampleTime=1e-08
  Product8 : Product  Inputs=**  OutDataTypeStr=fixdt(1, 48, 28)  SampleTime=1e-08
  Sqrt : Sqrt  OutputSignalType=real  SaturateOnIntegerOverflow=on
  StateControl : StateControl  StateControl=Synchronous
  Switch : Switch  Criteria=u2 ~= 0  Threshold=double(0)  OutDataTypeStr=fixdt(1, 73, 34)  SampleTime=1e-08
  Switch1 : Switch  Criteria=u2 ~= 0  Threshold=double(0)  OutDataTypeStr=fixdt(1, 73, 34)  SampleTime=1e-08
  c_out : Outport  InitialOutput=0
  sout_r : Outport  Port=2  InitialOutput=0
  sout_i : Outport  Port=3  InitialOutput=0
  rout_r : Outport  Port=4  InitialOutput=0
  rout_i : Outport  Port=5  InitialOutput=0
  wires:
  Enable/1 -> Delay6/Enable, Delay5/Enable, Delay4/Enable, Delay3/Enable, Delay2/Enable, Delay1/Enable
  uin_r/1 -> Product3/2, Product3/1, Delay3/1(in0)
  uin_i/1 -> Product4/2, Product4/1, Delay2/1(in0)
  En_bp/1 -> Switch1/2, Switch/2
  Bin_r/1 -> Product6/1
  Bin_i/1 -> Product7/1
  Add/1 -> Add1/1
  Add1/1 -> Sqrt/1
  Constant/1 -> Switch1/3
  Data Type Conversion2/1 -> rout_r/1
  Data Type Conversion3/1 -> Product8/2, Product8/1
  Data Type Conversion4/1 -> c_out/1
  Data Type Conversion5/1 -> sout_i/1
  Data Type Conversion7/1 -> sout_r/1
  Data Type Conversion8/1 -> rout_i/1
  Delay1/1(out0) -> Add1/2
  Delay2/1(out0) -> Product2/2
  Delay3/1(out0) -> Product5/2
  Delay4/1(out0) -> Product1/1
  Delay5/1(out0) -> Data Type Conversion2/1
  Delay6/1(out0) -> Data Type Conversion8/1
  HDL Reciprocal/1(Out1) -> Product7/2, Product6/2, Product5/1, Product2/1, Product1/2
  Product1/1 -> Data Type Conversion4/1
  Product2/1 -> Data Type Conversion5/1
  Product3/1 -> Add/1
  Product4/1 -> Add/2
  Product5/1 -> Data Type Conversion7/1
  Product6/1 -> Switch/1
  Product7/1 -> Switch1/1
  Product8/1 -> Delay1/1(in0)
  Sqrt/1 -> Switch/3, HDL Reciprocal/1(In1), Data Type Conversion3/1, Delay4/1(in0)
  Switch/1 -> Delay5/1(in0)
  Switch1/1 -> Delay6/1(in0)

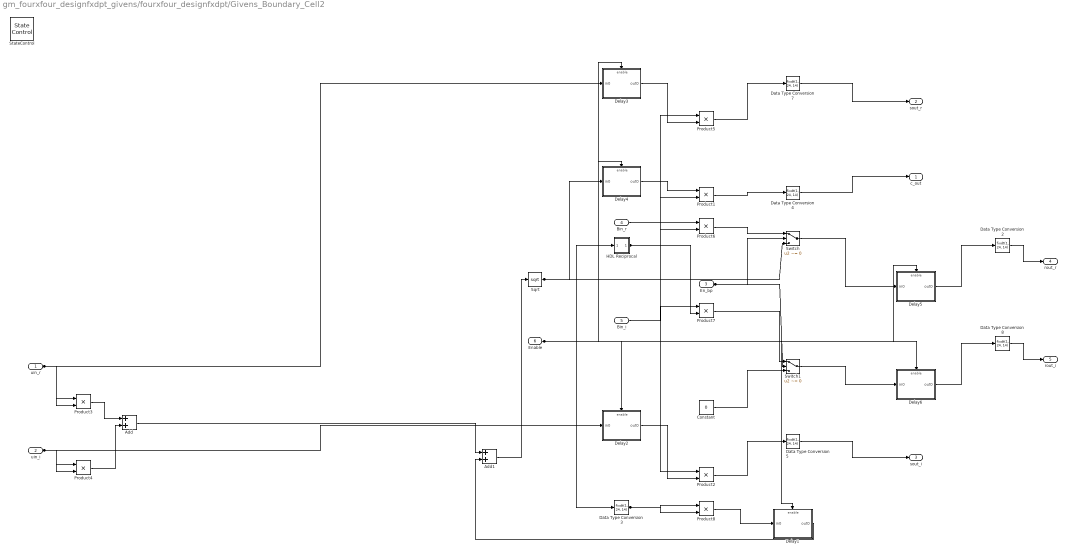
== system gm_fourxfour_designfxdpt_givens/fourxfour_designfxdpt/Givens_Boundary_Cell2 ==
  uin_r : Inport  OutDataTypeStr=fixdt(1, 24, 14)  SampleTime=1e-08
  uin_i : Inport  Port=2  OutDataTypeStr=fixdt(1, 24, 14)  SampleTime=1e-08
  En_bp : Inport  Port=3  OutDataTypeStr=boolean  SampleTime=1e-08
  Bin_r : Inport  Port=4  OutDataTypeStr=fixdt(1, 24, 14)  SampleTime=1e-08
  Bin_i : Inport  Port=5  OutDataTypeStr=fixdt(1, 24, 14)  SampleTime=1e-08
  Enable : Inport  Port=6  OutDataTypeStr=boolean  SampleTime=1e-08
  Add : Sum  AccumDataTypeStr=fixdt(1, 49, 28)  OutDataTypeStr=fixdt(1, 49, 28)  SampleTime=1e-08
  Add1 : Sum  AccumDataTypeStr=fixdt(1, 50, 28)  OutDataTypeStr=fixdt(0, 49, 28)  SampleTime=1e-08
  Constant : Constant  Value=0  OutDataTypeStr=fixdt(1, 24, 14)  SampleTime=-1
  Data Type Conversion{2..5,7..8} (6 alike) : DataTypeConversion  OutDataTypeStr=fixdt(1, 24, 14)  SampleTime=1e-08
  Delay1 : Subsystem
      settings: MinAlgLoopOccurrences=on
  Delay2 : Subsystem
      settings: MinAlgLoopOccurrences=on
  Delay3 : Subsystem
      settings: MinAlgLoopOccurrences=on
  Delay4 : Subsystem
      settings: MinAlgLoopOccurrences=on
  Delay5 : Subsystem
      settings: MinAlgLoopOccurrences=on
  Delay6 : Subsystem
      settings: MinAlgLoopOccurrences=on
  HDL Reciprocal : Subsystem
  Product1 : Product  Inputs=**  OutDataTypeStr=fixdt(0, 98, 48)  SampleTime=1e-08
  Product{2,5..7} (4 alike) : Product  Inputs=**  OutDataTypeStr=fixdt(1, 73, 34)  SampleTime=1e-08
  Product3 : Product  Inputs=**  OutDataTypeStr=fixdt(1, 48, 28)  SampleTime=1e-08
  Product4 : Product  Inputs=**  OutDataTypeStr=fixdt(1, 48, 28)  SampleTime=1e-08
  Product8 : Product  Inputs=**  OutDataTypeStr=fixdt(1, 48, 28)  SampleTime=1e-08
  Sqrt : Sqrt  OutputSignalType=real  SaturateOnIntegerOverflow=on
  StateControl : StateControl  StateControl=Synchronous
  Switch : Switch  Criteria=u2 ~= 0  Threshold=double(0)  OutDataTypeStr=fixdt(1, 73, 34)  SampleTime=1e-08
  Switch1 : Switch  Criteria=u2 ~= 0  Threshold=double(0)  OutDataTypeStr=fixdt(1, 73, 34)  SampleTime=1e-08
  c_out : Outport  InitialOutput=0
  sout_r : Outport  Port=2  InitialOutput=0
  sout_i : Outport  Port=3  InitialOutput=0
  rout_r : Outport  Port=4  InitialOutput=0
  rout_i : Outport  Port=5  InitialOutput=0
  wires:
  Enable/1 -> Delay6/Enable, Delay5/Enable, Delay4/Enable, Delay3/Enable, Delay2/Enable, Delay1/Enable
  uin_r/1 -> Product3/2, Product3/1, Delay3/1(in0)
  uin_i/1 -> Product4/2, Product4/1, Delay2/1(in0)
  En_bp/1 -> Switch1/2, Switch/2
  Bin_r/1 -> Product6/1
  Bin_i/1 -> Product7/1
  Add/1 -> Add1/1
  Add1/1 -> Sqrt/1
  Constant/1 -> Switch1/3
  Data Type Conversion2/1 -> rout_r/1
  Data Type Conversion3/1 -> Product8/2, Product8/1
  Data Type Conversion4/1 -> c_out/1
  Data Type Conversion5/1 -> sout_i/1
  Data Type Conversion7/1 -> sout_r/1
  Data Type Conversion8/1 -> rout_i/1
  Delay1/1(out0) -> Add1/2
  Delay2/1(out0) -> Product2/2
  Delay3/1(out0) -> Product5/2
  Delay4/1(out0) -> Product1/1
  Delay5/1(out0) -> Data Type Conversion2/1
  Delay6/1(out0) -> Data Type Conversion8/1
  HDL Reciprocal/1(Out1) -> Product7/2, Product6/2, Product5/1, Product2/1, Product1/2
  Product1/1 -> Data Type Conversion4/1
  Product2/1 -> Data Type Conversion5/1
  Product3/1 -> Add/1
  Product4/1 -> Add/2
  Product5/1 -> Data Type Conversion7/1
  Product6/1 -> Switch/1
  Product7/1 -> Switch1/1
  Product8/1 -> Delay1/1(in0)
  Sqrt/1 -> Switch/3, HDL Reciprocal/1(In1), Data Type Conversion3/1, Delay4/1(in0)
  Switch/1 -> Delay5/1(in0)
  Switch1/1 -> Delay6/1(in0)

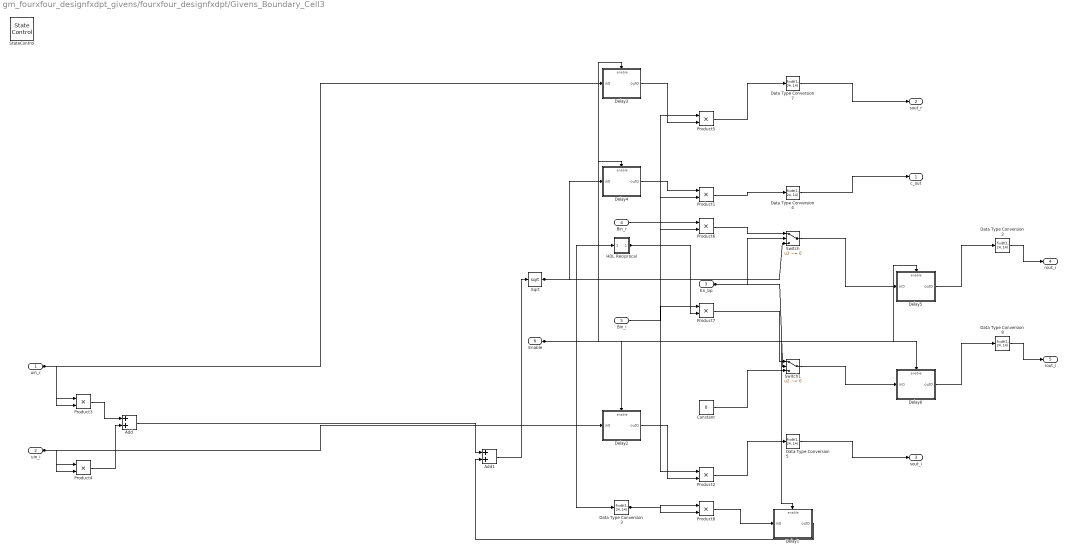
== system gm_fourxfour_designfxdpt_givens/fourxfour_designfxdpt/Givens_Boundary_Cell3 ==
  uin_r : Inport  OutDataTypeStr=fixdt(1, 24, 14)  SampleTime=1e-08
  uin_i : Inport  Port=2  OutDataTypeStr=fixdt(1, 24, 14)  SampleTime=1e-08
  En_bp : Inport  Port=3  OutDataTypeStr=boolean  SampleTime=1e-08
  Bin_r : Inport  Port=4  OutDataTypeStr=fixdt(1, 24, 14)  SampleTime=1e-08
  Bin_i : Inport  Port=5  OutDataTypeStr=fixdt(1, 24, 14)  SampleTime=1e-08
  Enable : Inport  Port=6  OutDataTypeStr=boolean  SampleTime=1e-08
  Add : Sum  AccumDataTypeStr=fixdt(1, 49, 28)  OutDataTypeStr=fixdt(1, 49, 28)  SampleTime=1e-08
  Add1 : Sum  AccumDataTypeStr=fixdt(1, 50, 28)  OutDataTypeStr=fixdt(0, 49, 28)  SampleTime=1e-08
  Constant : Constant  Value=0  OutDataTypeStr=fixdt(1, 24, 14)  SampleTime=-1
  Data Type Conversion{2..5,7..8} (6 alike) : DataTypeConversion  OutDataTypeStr=fixdt(1, 24, 14)  SampleTime=1e-08
  Delay1 : Subsystem
      settings: MinAlgLoopOccurrences=on
  Delay2 : Subsystem
      settings: MinAlgLoopOccurrences=on
  Delay3 : Subsystem
      settings: MinAlgLoopOccurrences=on
  Delay4 : Subsystem
      settings: MinAlgLoopOccurrences=on
  Delay5 : Subsystem
      settings: MinAlgLoopOccurrences=on
  Delay6 : Subsystem
      settings: MinAlgLoopOccurrences=on
  HDL Reciprocal : Subsystem
  Product1 : Product  Inputs=**  OutDataTypeStr=fixdt(0, 98, 48)  SampleTime=1e-08
  Product{2,5..7} (4 alike) : Product  Inputs=**  OutDataTypeStr=fixdt(1, 73, 34)  SampleTime=1e-08
  Product3 : Product  Inputs=**  OutDataTypeStr=fixdt(1, 48, 28)  SampleTime=1e-08
  Product4 : Product  Inputs=**  OutDataTypeStr=fixdt(1, 48, 28)  SampleTime=1e-08
  Product8 : Product  Inputs=**  OutDataTypeStr=fixdt(1, 48, 28)  SampleTime=1e-08
  Sqrt : Sqrt  OutputSignalType=real  SaturateOnIntegerOverflow=on
  StateControl : StateControl  StateControl=Synchronous
  Switch : Switch  Criteria=u2 ~= 0  Threshold=double(0)  OutDataTypeStr=fixdt(1, 73, 34)  SampleTime=1e-08
  Switch1 : Switch  Criteria=u2 ~= 0  Threshold=double(0)  OutDataTypeStr=fixdt(1, 73, 34)  SampleTime=1e-08
  c_out : Outport  InitialOutput=0
  sout_r : Outport  Port=2  InitialOutput=0
  sout_i : Outport  Port=3  InitialOutput=0
  rout_r : Outport  Port=4  InitialOutput=0
  rout_i : Outport  Port=5  InitialOutput=0
  wires:
  Enable/1 -> Delay6/Enable, Delay5/Enable, Delay4/Enable, Delay3/Enable, Delay2/Enable, Delay1/Enable
  uin_r/1 -> Product3/2, Product3/1, Delay3/1(in0)
  uin_i/1 -> Product4/2, Product4/1, Delay2/1(in0)
  En_bp/1 -> Switch1/2, Switch/2
  Bin_r/1 -> Product6/1
  Bin_i/1 -> Product7/1
  Add/1 -> Add1/1
  Add1/1 -> Sqrt/1
  Constant/1 -> Switch1/3
  Data Type Conversion2/1 -> rout_r/1
  Data Type Conversion3/1 -> Product8/2, Product8/1
  Data Type Conversion4/1 -> c_out/1
  Data Type Conversion5/1 -> sout_i/1
  Data Type Conversion7/1 -> sout_r/1
  Data Type Conversion8/1 -> rout_i/1
  Delay1/1(out0) -> Add1/2
  Delay2/1(out0) -> Product2/2
  Delay3/1(out0) -> Product5/2
  Delay4/1(out0) -> Product1/1
  Delay5/1(out0) -> Data Type Conversion2/1
  Delay6/1(out0) -> Data Type Conversion8/1
  HDL Reciprocal/1(Out1) -> Product7/2, Product6/2, Product5/1, Product2/1, Product1/2
  Product1/1 -> Data Type Conversion4/1
  Product2/1 -> Data Type Conversion5/1
  Product3/1 -> Add/1
  Product4/1 -> Add/2
  Product5/1 -> Data Type Conversion7/1
  Product6/1 -> Switch/1
  Product7/1 -> Switch1/1
  Product8/1 -> Delay1/1(in0)
  Sqrt/1 -> Switch/3, HDL Reciprocal/1(In1), Data Type Conversion3/1, Delay4/1(in0)
  Switch/1 -> Delay5/1(in0)
  Switch1/1 -> Delay6/1(in0)

== system gm_fourxfour_designfxdpt_givens/fourxfour_designfxdpt/Givens_Internal_BW_Cell ==
  uin_r : Inport  OutDataTypeStr=fixdt(1, 24, 14)  SampleTime=1e-08
  uin_i : Inport  Port=2  OutDataTypeStr=fixdt(1, 24, 14)  SampleTime=1e-08
  cin : Inport  Port=3  OutDataTypeStr=fixdt(1, 24, 14)  SampleTime=1e-08
  sin_r : Inport  Port=4  OutDataTypeStr=fixdt(1, 24, 14)  SampleTime=1e-08
  sin_i : Inport  Port=5  OutDataTypeStr=fixdt(1, 24, 14)  SampleTime=1e-08
  Enable : Inport  Port=6  OutDataTypeStr=boolean  SampleTime=1e-08
  Add : Sum  Inputs=+-  AccumDataTypeStr=fixdt(1, 50, 28)  OutDataTypeStr=fixdt(1, 50, 28)  SampleTime=1e-08
  Add1 : Sum  Inputs=+-  AccumDataTypeStr=fixdt(1, 50, 28)  OutDataTypeStr=fixdt(1, 50, 28)  SampleTime=1e-08
  Data Type Conversion{8..11} (4 alike) : DataTypeConversion  OutDataTypeStr=fixdt(1, 24, 14)  SampleTime=1e-08
  Delay : Subsystem
      settings: MinAlgLoopOccurrences=on
  Delay1 : Subsystem
      settings: MinAlgLoopOccurrences=on
  StateControl : StateControl  StateControl=Synchronous
  Unary Minus : UnaryMinus  SampleTime=1e-08
  c*r_i : Product  Inputs=**  OutDataTypeStr=fixdt(1, 48, 28)  SampleTime=1e-08
  c*r_r : Product  Inputs=**  OutDataTypeStr=fixdt(1, 48, 28)  SampleTime=1e-08
  c*uin_i : Product  Inputs=**  OutDataTypeStr=fixdt(1, 48, 28)  SampleTime=1e-08
  c*uin_r : Product  Inputs=**  OutDataTypeStr=fixdt(1, 48, 28)  SampleTime=1e-08
  complex_mul : Subsystem
  complex_mul1 : Subsystem
  r_im : Sum  AccumDataTypeStr=fixdt(1, 50, 28)  OutDataTypeStr=fixdt(1, 50, 28)  SampleTime=1e-08
  r_r : Sum  AccumDataTypeStr=fixdt(1, 50, 28)  OutDataTypeStr=fixdt(1, 50, 28)  SampleTime=1e-08
  uout_r : Outport  InitialOutput=0
  uout_i : Outport  Port=2  InitialOutput=0
  cout : Outport  Port=3  InitialOutput=0
  sout_r : Outport  Port=4  InitialOutput=0
  sout_i : Outport  Port=5  InitialOutput=0
  rout_i : Outport  Port=6  InitialOutput=0
  rout_r : Outport  Port=7  InitialOutput=0
  wires:
  Enable/1 -> Delay1/Enable, Delay/Enable
  uin_r/1 -> c*uin_r/2, complex_mul1/3(In2_r)
  uin_i/1 -> c*uin_i/2, complex_mul1/4(In2_i)
  cin/1 -> c*uin_r/1, c*uin_i/1, c*r_r/1, c*r_i/1, cout/1
  sin_r/1 -> complex_mul/1(In1_r), complex_mul1/1(In1_r), sout_r/1
  sin_i/1 -> Unary Minus/1, complex_mul/2(In1_i), sout_i/1
  Add/1 -> Data Type Conversion10/1
  Add1/1 -> Data Type Conversion11/1
  Data Type Conversion10/1 -> uout_r/1
  Data Type Conversion11/1 -> uout_i/1
  Data Type Conversion8/1 -> Delay/1(in0), rout_i/1
  Data Type Conversion9/1 -> Delay1/1(in0), rout_r/1
  Delay/1(out0) -> c*r_i/2, complex_mul/4(In2_i)
  Delay1/1(out0) -> c*r_r/2, complex_mul/3(In2_r)
  Unary Minus/1 -> complex_mul1/2(In1_i)
  c*r_i/1 -> r_im/2
  c*r_r/1 -> r_r/2
  c*uin_i/1 -> Add1/1
  c*uin_r/1 -> Add/1
  complex_mul/1(Out1_r) -> Add/2
  complex_mul/2(Out1_i) -> Add1/2
  complex_mul1/1(Out1_r) -> r_r/1
  complex_mul1/2(Out1_i) -> r_im/1
  r_im/1 -> Data Type Conversion8/1
  r_r/1 -> Data Type Conversion9/1

== system gm_fourxfour_designfxdpt_givens/fourxfour_designfxdpt/Givens_Internal_BW_Cell1 ==
  uin_r : Inport  OutDataTypeStr=fixdt(1, 24, 14)  SampleTime=1e-08
  uin_i : Inport  Port=2  OutDataTypeStr=fixdt(1, 24, 14)  SampleTime=1e-08
  cin : Inport  Port=3  OutDataTypeStr=fixdt(1, 24, 14)  SampleTime=1e-08
  sin_r : Inport  Port=4  OutDataTypeStr=fixdt(1, 24, 14)  SampleTime=1e-08
  sin_i : Inport  Port=5  OutDataTypeStr=fixdt(1, 24, 14)  SampleTime=1e-08
  Enable : Inport  Port=6  OutDataTypeStr=boolean  SampleTime=1e-08
  Add : Sum  Inputs=+-  AccumDataTypeStr=fixdt(1, 50, 28)  OutDataTypeStr=fixdt(1, 50, 28)  SampleTime=1e-08
  Add1 : Sum  Inputs=+-  AccumDataTypeStr=fixdt(1, 50, 28)  OutDataTypeStr=fixdt(1, 50, 28)  SampleTime=1e-08
  Data Type Conversion{8..11} (4 alike) : DataTypeConversion  OutDataTypeStr=fixdt(1, 24, 14)  SampleTime=1e-08
  Delay : Subsystem
      settings: MinAlgLoopOccurrences=on
  Delay1 : Subsystem
      settings: MinAlgLoopOccurrences=on
  StateControl : StateControl  StateControl=Synchronous
  Unary Minus : UnaryMinus  SampleTime=1e-08
  c*r_i : Product  Inputs=**  OutDataTypeStr=fixdt(1, 48, 28)  SampleTime=1e-08
  c*r_r : Product  Inputs=**  OutDataTypeStr=fixdt(1, 48, 28)  SampleTime=1e-08
  c*uin_i : Product  Inputs=**  OutDataTypeStr=fixdt(1, 48, 28)  SampleTime=1e-08
  c*uin_r : Product  Inputs=**  OutDataTypeStr=fixdt(1, 48, 28)  SampleTime=1e-08
  complex_mul : Subsystem
  complex_mul1 : Subsystem
  r_im : Sum  AccumDataTypeStr=fixdt(1, 50, 28)  OutDataTypeStr=fixdt(1, 50, 28)  SampleTime=1e-08
  r_r : Sum  AccumDataTypeStr=fixdt(1, 50, 28)  OutDataTypeStr=fixdt(1, 50, 28)  SampleTime=1e-08
  uout_r : Outport  InitialOutput=0
  uout_i : Outport  Port=2  InitialOutput=0
  cout : Outport  Port=3  InitialOutput=0
  sout_r : Outport  Port=4  InitialOutput=0
  sout_i : Outport  Port=5  InitialOutput=0
  rout_i : Outport  Port=6  InitialOutput=0
  rout_r : Outport  Port=7  InitialOutput=0
  wires:
  Enable/1 -> Delay1/Enable, Delay/Enable
  uin_r/1 -> c*uin_r/2, complex_mul1/3(In2_r)
  uin_i/1 -> c*uin_i/2, complex_mul1/4(In2_i)
  cin/1 -> c*uin_r/1, c*uin_i/1, c*r_r/1, c*r_i/1, cout/1
  sin_r/1 -> complex_mul/1(In1_r), complex_mul1/1(In1_r), sout_r/1
  sin_i/1 -> Unary Minus/1, complex_mul/2(In1_i), sout_i/1
  Add/1 -> Data Type Conversion10/1
  Add1/1 -> Data Type Conversion11/1
  Data Type Conversion10/1 -> uout_r/1
  Data Type Conversion11/1 -> uout_i/1
  Data Type Conversion8/1 -> Delay/1(in0), rout_i/1
  Data Type Conversion9/1 -> Delay1/1(in0), rout_r/1
  Delay/1(out0) -> c*r_i/2, complex_mul/4(In2_i)
  Delay1/1(out0) -> c*r_r/2, complex_mul/3(In2_r)
  Unary Minus/1 -> complex_mul1/2(In1_i)
  c*r_i/1 -> r_im/2
  c*r_r/1 -> r_r/2
  c*uin_i/1 -> Add1/1
  c*uin_r/1 -> Add/1
  complex_mul/1(Out1_r) -> Add/2
  complex_mul/2(Out1_i) -> Add1/2
  complex_mul1/1(Out1_r) -> r_r/1
  complex_mul1/2(Out1_i) -> r_im/1
  r_im/1 -> Data Type Conversion8/1
  r_r/1 -> Data Type Conversion9/1

== system gm_fourxfour_designfxdpt_givens/fourxfour_designfxdpt/Givens_Internal_BW_Cell2 ==
  uin_r : Inport  OutDataTypeStr=fixdt(1, 24, 14)  SampleTime=1e-08
  uin_i : Inport  Port=2  OutDataTypeStr=fixdt(1, 24, 14)  SampleTime=1e-08
  cin : Inport  Port=3  OutDataTypeStr=fixdt(1, 24, 14)  SampleTime=1e-08
  sin_r : Inport  Port=4  OutDataTypeStr=fixdt(1, 24, 14)  SampleTime=1e-08
  sin_i : Inport  Port=5  OutDataTypeStr=fixdt(1, 24, 14)  SampleTime=1e-08
  Enable : Inport  Port=6  OutDataTypeStr=boolean  SampleTime=1e-08
  Add : Sum  Inputs=+-  AccumDataTypeStr=fixdt(1, 50, 28)  OutDataTypeStr=fixdt(1, 50, 28)  SampleTime=1e-08
  Add1 : Sum  Inputs=+-  AccumDataTypeStr=fixdt(1, 50, 28)  OutDataTypeStr=fixdt(1, 50, 28)  SampleTime=1e-08
  Data Type Conversion{8..11} (4 alike) : DataTypeConversion  OutDataTypeStr=fixdt(1, 24, 14)  SampleTime=1e-08
  Delay : Subsystem
      settings: MinAlgLoopOccurrences=on
  Delay1 : Subsystem
      settings: MinAlgLoopOccurrences=on
  StateControl : StateControl  StateControl=Synchronous
  Unary Minus : UnaryMinus  SampleTime=1e-08
  c*r_i : Product  Inputs=**  OutDataTypeStr=fixdt(1, 48, 28)  SampleTime=1e-08
  c*r_r : Product  Inputs=**  OutDataTypeStr=fixdt(1, 48, 28)  SampleTime=1e-08
  c*uin_i : Product  Inputs=**  OutDataTypeStr=fixdt(1, 48, 28)  SampleTime=1e-08
  c*uin_r : Product  Inputs=**  OutDataTypeStr=fixdt(1, 48, 28)  SampleTime=1e-08
  complex_mul : Subsystem
  complex_mul1 : Subsystem
  r_im : Sum  AccumDataTypeStr=fixdt(1, 50, 28)  OutDataTypeStr=fixdt(1, 50, 28)  SampleTime=1e-08
  r_r : Sum  AccumDataTypeStr=fixdt(1, 50, 28)  OutDataTypeStr=fixdt(1, 50, 28)  SampleTime=1e-08
  uout_r : Outport  InitialOutput=0
  uout_i : Outport  Port=2  InitialOutput=0
  cout : Outport  Port=3  InitialOutput=0
  sout_r : Outport  Port=4  InitialOutput=0
  sout_i : Outport  Port=5  InitialOutput=0
  rout_i : Outport  Port=6  InitialOutput=0
  rout_r : Outport  Port=7  InitialOutput=0
  wires:
  Enable/1 -> Delay1/Enable, Delay/Enable
  uin_r/1 -> c*uin_r/2, complex_mul1/3(In2_r)
  uin_i/1 -> c*uin_i/2, complex_mul1/4(In2_i)
  cin/1 -> c*uin_r/1, c*uin_i/1, c*r_r/1, c*r_i/1, cout/1
  sin_r/1 -> complex_mul/1(In1_r), complex_mul1/1(In1_r), sout_r/1
  sin_i/1 -> Unary Minus/1, complex_mul/2(In1_i), sout_i/1
  Add/1 -> Data Type Conversion10/1
  Add1/1 -> Data Type Conversion11/1
  Data Type Conversion10/1 -> uout_r/1
  Data Type Conversion11/1 -> uout_i/1
  Data Type Conversion8/1 -> Delay/1(in0), rout_i/1
  Data Type Conversion9/1 -> Delay1/1(in0), rout_r/1
  Delay/1(out0) -> c*r_i/2, complex_mul/4(In2_i)
  Delay1/1(out0) -> c*r_r/2, complex_mul/3(In2_r)
  Unary Minus/1 -> complex_mul1/2(In1_i)
  c*r_i/1 -> r_im/2
  c*r_r/1 -> r_r/2
  c*uin_i/1 -> Add1/1
  c*uin_r/1 -> Add/1
  complex_mul/1(Out1_r) -> Add/2
  complex_mul/2(Out1_i) -> Add1/2
  complex_mul1/1(Out1_r) -> r_r/1
  complex_mul1/2(Out1_i) -> r_im/1
  r_im/1 -> Data Type Conversion8/1
  r_r/1 -> Data Type Conversion9/1

== system gm_fourxfour_designfxdpt_givens/fourxfour_designfxdpt/Givens_Internal_BW_Cell3 ==
  uin_r : Inport  OutDataTypeStr=fixdt(1, 24, 14)  SampleTime=1e-08
  uin_i : Inport  Port=2  OutDataTypeStr=fixdt(1, 24, 14)  SampleTime=1e-08
  cin : Inport  Port=3  OutDataTypeStr=fixdt(1, 24, 14)  SampleTime=1e-08
  sin_r : Inport  Port=4  OutDataTypeStr=fixdt(1, 24, 14)  SampleTime=1e-08
  sin_i : Inport  Port=5  OutDataTypeStr=fixdt(1, 24, 14)  SampleTime=1e-08
  Enable : Inport  Port=6  OutDataTypeStr=boolean  SampleTime=1e-08
  Add : Sum  Inputs=+-  AccumDataTypeStr=fixdt(1, 50, 28)  OutDataTypeStr=fixdt(1, 50, 28)  SampleTime=1e-08
  Add1 : Sum  Inputs=+-  AccumDataTypeStr=fixdt(1, 50, 28)  OutDataTypeStr=fixdt(1, 50, 28)  SampleTime=1e-08
  Data Type Conversion{8..11} (4 alike) : DataTypeConversion  OutDataTypeStr=fixdt(1, 24, 14)  SampleTime=1e-08
  Delay : Subsystem
      settings: MinAlgLoopOccurrences=on
  Delay1 : Subsystem
      settings: MinAlgLoopOccurrences=on
  StateControl : StateControl  StateControl=Synchronous
  Unary Minus : UnaryMinus  SampleTime=1e-08
  c*r_i : Product  Inputs=**  OutDataTypeStr=fixdt(1, 48, 28)  SampleTime=1e-08
  c*r_r : Product  Inputs=**  OutDataTypeStr=fixdt(1, 48, 28)  SampleTime=1e-08
  c*uin_i : Product  Inputs=**  OutDataTypeStr=fixdt(1, 48, 28)  SampleTime=1e-08
  c*uin_r : Product  Inputs=**  OutDataTypeStr=fixdt(1, 48, 28)  SampleTime=1e-08
  complex_mul : Subsystem
  complex_mul1 : Subsystem
  r_im : Sum  AccumDataTypeStr=fixdt(1, 50, 28)  OutDataTypeStr=fixdt(1, 50, 28)  SampleTime=1e-08
  r_r : Sum  AccumDataTypeStr=fixdt(1, 50, 28)  OutDataTypeStr=fixdt(1, 50, 28)  SampleTime=1e-08
  uout_r : Outport  InitialOutput=0
  uout_i : Outport  Port=2  InitialOutput=0
  cout : Outport  Port=3  InitialOutput=0
  sout_r : Outport  Port=4  InitialOutput=0
  sout_i : Outport  Port=5  InitialOutput=0
  rout_i : Outport  Port=6  InitialOutput=0
  rout_r : Outport  Port=7  InitialOutput=0
  wires:
  Enable/1 -> Delay1/Enable, Delay/Enable
  uin_r/1 -> c*uin_r/2, complex_mul1/3(In2_r)
  uin_i/1 -> c*uin_i/2, complex_mul1/4(In2_i)
  cin/1 -> c*uin_r/1, c*uin_i/1, c*r_r/1, c*r_i/1, cout/1
  sin_r/1 -> complex_mul/1(In1_r), complex_mul1/1(In1_r), sout_r/1
  sin_i/1 -> Unary Minus/1, complex_mul/2(In1_i), sout_i/1
  Add/1 -> Data Type Conversion10/1
  Add1/1 -> Data Type Conversion11/1
  Data Type Conversion10/1 -> uout_r/1
  Data Type Conversion11/1 -> uout_i/1
  Data Type Conversion8/1 -> Delay/1(in0), rout_i/1
  Data Type Conversion9/1 -> Delay1/1(in0), rout_r/1
  Delay/1(out0) -> c*r_i/2, complex_mul/4(In2_i)
  Delay1/1(out0) -> c*r_r/2, complex_mul/3(In2_r)
  Unary Minus/1 -> complex_mul1/2(In1_i)
  c*r_i/1 -> r_im/2
  c*r_r/1 -> r_r/2
  c*uin_i/1 -> Add1/1
  c*uin_r/1 -> Add/1
  complex_mul/1(Out1_r) -> Add/2
  complex_mul/2(Out1_i) -> Add1/2
  complex_mul1/1(Out1_r) -> r_r/1
  complex_mul1/2(Out1_i) -> r_im/1
  r_im/1 -> Data Type Conversion8/1
  r_r/1 -> Data Type Conversion9/1
